simulink model "generalized_plant"  (R2024b)
settings: Solver=VariableStepAuto  StartTime=0.0  StopTime=10.0  RelTol=1e-3
values from neighbouring files (symbols this model uses):
  Ga = 1    [p21.m]
  Gf = 1/(Gs*Kd)    (= 0.0666666666667)    [p21.m]
  Gs = 5    [p21.m]
libraries: cstblocks x3
settings Model: Creator=aayan  LastModifiedBy=aayan

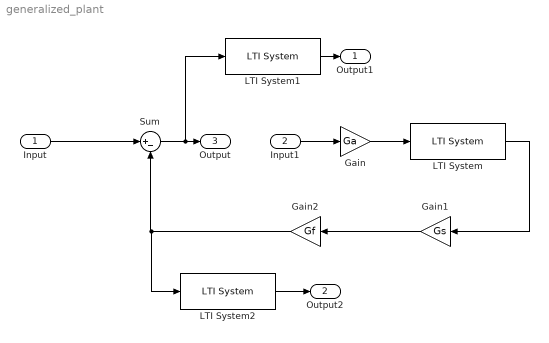
== system generalized_plant ==
  Input : Inport
  Input1 : Inport  Port=2
  Gain : Gain  Gain=Ga
  Gain1 : Gain  Gain=Gs
  Gain2 : Gain  Gain=Gf
  LTI System : cstblocks/LTI System  sys=Gpn  IC=[]  PadeOrder=0
  LTI System1 : cstblocks/LTI System  sys=W1mod  IC=[]  PadeOrder=0
  LTI System2 : cstblocks/LTI System  sys=W2mod  IC=[]  PadeOrder=0
  Sum : Sum  Inputs=|+-
  Output1 : Outport
  Output2 : Outport  Port=2
  Output : Outport  Port=3
  wires:
  Input/1 -> Sum/1
  Sum/1 -> LTI System1/1, Output/1
  Input1/1 -> Gain/1
  Gain/1 -> LTI System/1
  Gain1/1 -> Gain2/1
  LTI System/1 -> Gain1/1
  Gain2/1 -> LTI System2/1, Sum/2
  LTI System1/1 -> Output1/1
  LTI System2/1 -> Output2/1
